simulink model "ME486C_Dyno_DAQ_Test_Version"  (R2025a)
settings: Solver=FixedStepDiscrete  StartTime=0.0  StopTime=20.0  FixedStep=0.02  RelTol=1e-3
undefined symbols (not defined in the file): Flow_initial, Flow_slope, Force_initial, Force_slope, RPM_initial, RPM_slope, Tin_initial, Tin_slope, Tout_slope
libraries: simulink x8
settings Model: Creator=YHQ  LastModifiedBy=YHQ

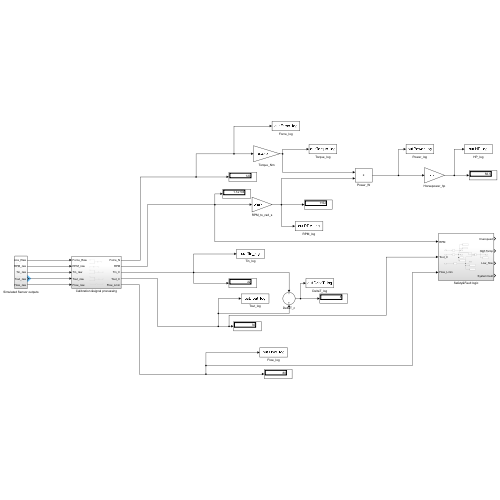
[thumbnail: Simulink's stored preview of the top-level diagram]
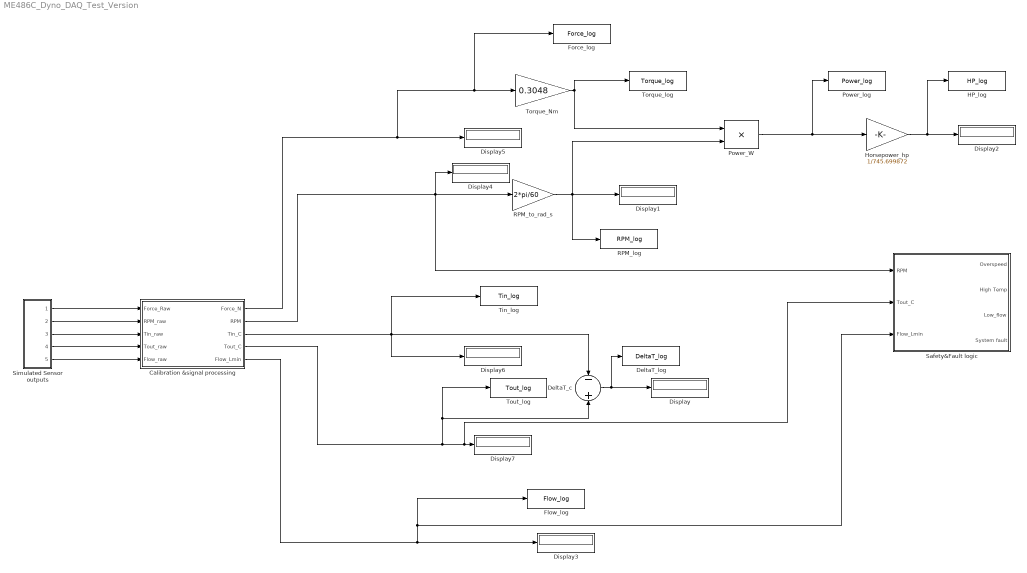
== system ME486C_Dyno_DAQ_Test_Version ==
  Calibration &signal processing : Subsystem
  DeltaT_c : Sum  Inputs=-+
  DeltaT_log : ToWorkspace  VariableName=DeltaT_log  SaveFormat=Timeseries  SampleTime=-1
  Display{,1..7} (8 alike) : Display
  Flow_log : ToWorkspace  VariableName=Flow_log  SaveFormat=Timeseries  SampleTime=-1
  Force_log : ToWorkspace  VariableName=Force_log  SaveFormat=Timeseries  SampleTime=-1
  HP_log : ToWorkspace  VariableName=HP_log  SaveFormat=Timeseries  SampleTime=-1
  Horsepower_hp : Gain  Gain=1/745.699872
  Power_W : Product
  Power_log : ToWorkspace  VariableName=Power_log  SaveFormat=Timeseries  SampleTime=-1
  RPM_log : ToWorkspace  VariableName=RPM_log  SaveFormat=Timeseries  SampleTime=-1
  RPM_to_rad_s : Gain  Gain=2*pi/60
  Safety&Fault logic : Subsystem
  Simulated Sensor outputs : Subsystem
  Tin_log : ToWorkspace  VariableName=Tin_log  SaveFormat=Timeseries  SampleTime=-1
  Torque_Nm : Gain  Gain=0.3048
  Torque_log : ToWorkspace  VariableName=Torque_log  SaveFormat=Timeseries  SampleTime=-1
  Tout_log : ToWorkspace  VariableName=Tout_log  SaveFormat=Timeseries  SampleTime=-1
  wires:
  RPM_to_rad_s/1 -> RPM_log/1, Power_W/2, Display1/1
  Torque_Nm/1 -> Torque_log/1, Power_W/1
  Power_W/1 -> Power_log/1, Horsepower_hp/1
  Horsepower_hp/1 -> Display2/1, HP_log/1
  DeltaT_c/1 -> DeltaT_log/1, Display/1
  Simulated Sensor outputs/1(Force_Raw) -> Calibration &signal processing/1(Force_Raw)
  Simulated Sensor outputs/2(RPM_raw) -> Calibration &signal processing/2(RPM_raw)
  Simulated Sensor outputs/3(Tin_raw) -> Calibration &signal processing/3(Tin_raw)
  Simulated Sensor outputs/4(Tout_raw) -> Calibration &signal processing/4(Tout_raw)
  Simulated Sensor outputs/5(Flow_raw) -> Calibration &signal processing/5(Flow_raw)
  Calibration &signal processing/1(Force_N) -> Force_log/1, Torque_Nm/1, Display5/1
  Calibration &signal processing/2(RPM) -> Safety&Fault logic/1(RPM), Display4/1, RPM_to_rad_s/1
  Calibration &signal processing/3(Tin_C) -> DeltaT_c/1, Display6/1, Tin_log/1
  Calibration &signal processing/4(Tout_C) -> DeltaT_c/2, Tout_log/1, Safety&Fault logic/2(Tout_C), Display7/1
  Calibration &signal processing/5(Flow_Lmin) -> Flow_log/1, Safety&Fault logic/3(Flow_Lmin), Display3/1

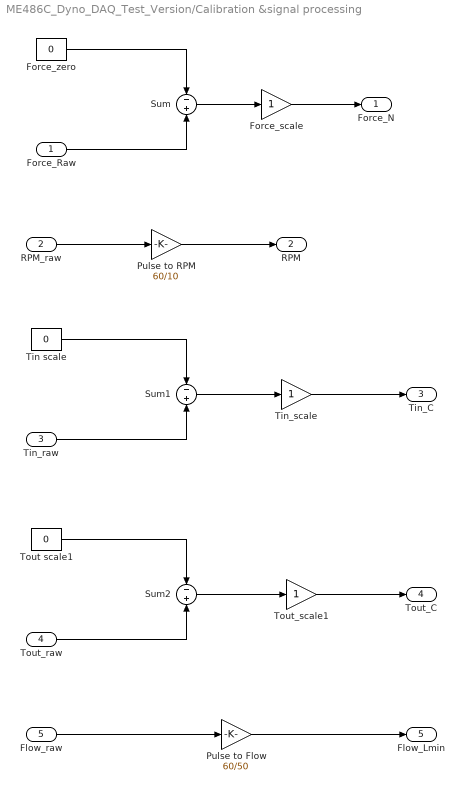
== system ME486C_Dyno_DAQ_Test_Version/Calibration &signal processing ==
  Force_Raw : Inport
  RPM_raw : Inport  Port=2
  Tin_raw : Inport  Port=3
  Tout_raw : Inport  Port=4
  Flow_raw : Inport  Port=5
  Force_scale : Gain
  Force_zero : Constant  Value=0
  Pulse to Flow : Gain  Gain=60/50
  Pulse to RPM : Gain  Gain=60/10
  Sum : Sum  Inputs=-+
  Sum1 : Sum  Inputs=-+
  Sum2 : Sum  Inputs=-+
  Tin scale : Constant  Value=0
  Tin_scale : Gain
  Tout scale1 : Constant  Value=0
  Tout_scale1 : Gain
  Force_N : Outport
  RPM : Outport  Port=2
  Tin_C : Outport  Port=3
  Tout_C : Outport  Port=4
  Flow_Lmin : Outport  Port=5
  wires:
  Force_zero/1 -> Sum/1
  Force_Raw/1 -> Sum/2
  Sum/1 -> Force_scale/1
  Force_scale/1 -> Force_N/1
  RPM_raw/1 -> Pulse to RPM/1
  Pulse to RPM/1 -> RPM/1
  Tin_scale/1 -> Tin_C/1
  Tin_raw/1 -> Sum1/2
  Sum1/1 -> Tin_scale/1
  Tin scale/1 -> Sum1/1
  Tout_raw/1 -> Sum2/2
  Tout scale1/1 -> Sum2/1
  Sum2/1 -> Tout_scale1/1
  Tout_scale1/1 -> Tout_C/1
  Flow_raw/1 -> Pulse to Flow/1
  Pulse to Flow/1 -> Flow_Lmin/1

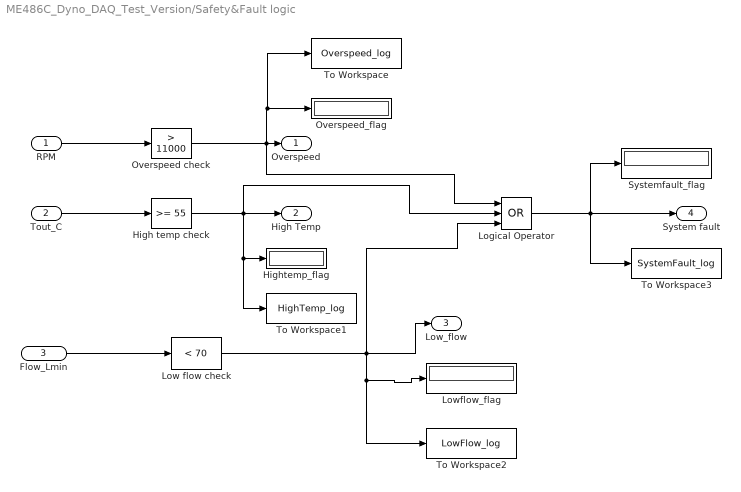
== system ME486C_Dyno_DAQ_Test_Version/Safety&Fault logic ==
  RPM : Inport
  Tout_C : Inport  Port=2
  Flow_Lmin : Inport  Port=3
  High temp check : simulink/Logic and Bit Operations/Compare To Constant  relop=>=  const=55  OutDataTypeStr=boolean
  Hightemp_flag : Display
  Logical Operator : Logic  Operator=OR  Inputs=3  AllPortsSameDT=off  OutDataTypeStr=boolean
  Low flow check : simulink/Logic and Bit Operations/Compare To Constant  relop=<  const=70  OutDataTypeStr=boolean
  Lowflow_flag : Display
  Overspeed check : simulink/Logic and Bit Operations/Compare To Constant  relop=>  const=11000  OutDataTypeStr=boolean
  Overspeed_flag : Display
  Systemfault_flag : Display
  To Workspace : ToWorkspace  VariableName=Overspeed_log  SaveFormat=Timeseries  SampleTime=-1
  To Workspace1 : ToWorkspace  VariableName=HighTemp_log  SaveFormat=Timeseries  SampleTime=-1
  To Workspace2 : ToWorkspace  VariableName=LowFlow_log  SaveFormat=Timeseries  SampleTime=-1
  To Workspace3 : ToWorkspace  VariableName=SystemFault_log  SaveFormat=Timeseries  SampleTime=-1
  Overspeed : Outport
  High Temp : Outport  Port=2
  Low_flow : Outport  Port=3
  System fault : Outport  Port=4
  wires:
  Tout_C/1 -> High temp check/1
  RPM/1 -> Overspeed check/1
  Overspeed check/1 -> To Workspace/1, Overspeed_flag/1, Logical Operator/1, Overspeed/1
  High temp check/1 -> To Workspace1/1, Hightemp_flag/1, Logical Operator/2, High Temp/1
  Low flow check/1 -> Logical Operator/3, Low_flow/1, To Workspace2/1, Lowflow_flag/1
  Flow_Lmin/1 -> Low flow check/1
  Logical Operator/1 -> To Workspace3/1, Systemfault_flag/1, System fault/1

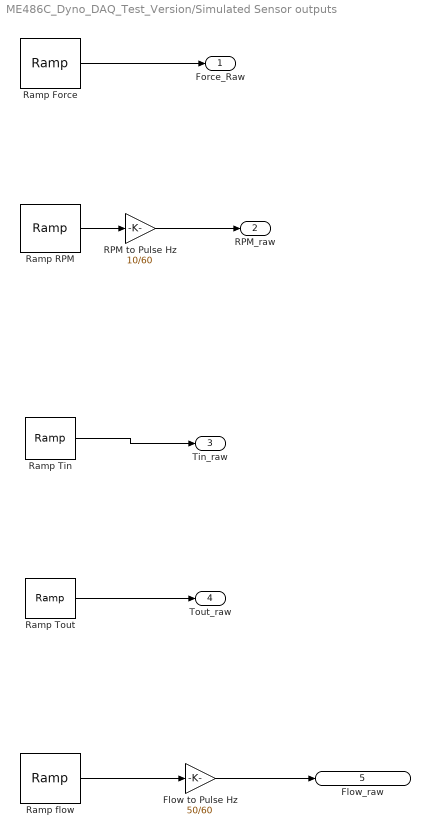
== system ME486C_Dyno_DAQ_Test_Version/Simulated Sensor outputs ==
  Flow to Pulse Hz : Gain  Gain=50/60
  RPM to Pulse Hz : Gain  Gain=10/60
  Ramp Force : simulink/Sources/Ramp  slope=Force_slope  start=0  InitialOutput=Force_initial
  Ramp RPM : simulink/Sources/Ramp  slope=RPM_slope  start=0  InitialOutput=RPM_initial
  Ramp Tin : simulink/Sources/Ramp  slope=Tin_slope  start=0  InitialOutput=Tin_initial
  Ramp Tout : simulink/Sources/Ramp  slope=Tout_slope  start=0  InitialOutput=Tin_initial
  Ramp flow : simulink/Sources/Ramp  slope=Flow_slope  start=0  InitialOutput=Flow_initial
  Force_Raw : Outport
  RPM_raw : Outport  Port=2
  Tin_raw : Outport  Port=3
  Tout_raw : Outport  Port=4
  Flow_raw : Outport  Port=5
  wires:
  Ramp Tout/1 -> Tout_raw/1
  Ramp Tin/1 -> Tin_raw/1
  Ramp Force/1 -> Force_Raw/1
  RPM to Pulse Hz/1 -> RPM_raw/1
  Ramp RPM/1 -> RPM to Pulse Hz/1
  Flow to Pulse Hz/1 -> Flow_raw/1
  Ramp flow/1 -> Flow to Pulse Hz/1
